simulink model "Model_3a_2015a"  (R2015a)
settings: Solver=ode45  StartTime=0.0  StopTime=10  RelTol=1e-3
undefined symbols (not defined in the file): c1, c2, K1, K2, K3, p1, Ts, wave
settings Model: CovModelRefEnable=off  Creator=s3blanch  LastModifiedBy=s3blanch
settings DataIOCC: SaveFormat=StructureWithTime
settings HardwareCC: ProdBitPerPointer=64  ProdLargestAtomicFloat=Float  ProdIntDivRoundTo=Zero  ProdEndianess=LittleEndian  ProdHWDeviceType=Specified
settings GRTTargetCC: GeneratePreprocessorConditionals=Use local settings

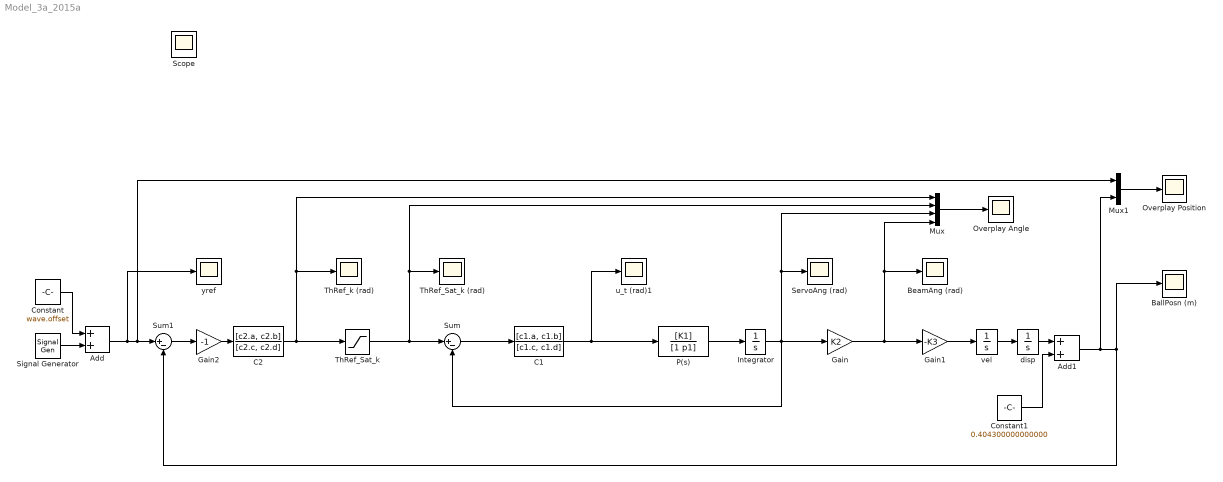
== system Model_3a_2015a ==
  " BeamAng (rad)" : Scope
      settings: YMin=-0.03886  YMax=0.03886  SaveName=BeamAng
  Add : Sum
  Add1 : Sum
  BallPosn (m) : Scope
      settings: YMin=-0.03732  YMax=0.33589  SaveName=BallPosn
  C1 : DiscreteTransferFcn  Numerator=[c1.a, c1.b]  Denominator=[c1.c, c1.d]  SampleTime=Ts
  C2 : DiscreteTransferFcn  Numerator=[c2.a, c2.b]  Denominator=[c2.c, c2.d]  SampleTime=Ts
  Constant : Constant  Value=wave.offset
  Constant1 : Constant  Value=0.404300000000000
  Gain : Gain  Gain=K2
  Gain1 : Gain  Gain=-K3
  Gain2 : Gain  Gain=-1
  Integrator : Integrator
  Mux : Mux
  Mux1 : Mux  Inputs=2
  Overplay Angle : Scope
      settings: TimeRange=25  YMin=-1.05154  YMax=1.20456
  Overplay Position : Scope
      settings: TimeRange=25  YMin=-0.03732  YMax=0.33589
  P(s) : TransferFcn  Numerator=[K1]  Denominator=[1 p1]
  ServoAng (rad) : Scope
      settings: YMin=-0.63804  YMax=0.63804  SaveName=ServoAng
  Signal Generator : SignalGenerator  WaveForm=square  Amplitude=-wave.amp  Frequency=0.2
  Sum : Sum  Inputs=|+-
  Sum1 : Sum  Inputs=|+-
  ThRef_Sat_k : Saturate  UpperLimit=0.7  LowerLimit=-0.7
  ThRef_Sat_k (rad) : Scope
      settings: YMin=-0.875  YMax=0.875  SaveName=ThRef
  ThRef_k (rad) : Scope
      settings: YMin=-1.05154  YMax=1.20456  SaveName=ref
  disp : Integrator
  u_t (rad)1 : Scope
      settings: YMin=-3.50155  YMax=2.92902  SaveName=u
  vel : Integrator
  yref : Scope
      settings: YMin=0.1275  YMax=0.2525  SaveName=yref
  Scope : Scope
      settings: YMin=-0.70238  YMax=0.70238
  wires:
  P(s)/1 -> Integrator/1
  Integrator/1 -> Gain/1, Sum/2, Mux/3, ServoAng (rad)/1
  Mux/1 -> Overplay Angle/1
  Sum/1 -> C1/1
  C1/1 -> P(s)/1, u_t (rad)1/1
  Gain1/1 -> vel/1
  vel/1 -> disp/1
  C2/1 -> Mux/1, ThRef_k (rad)/1, ThRef_Sat_k/1
  Mux1/1 -> Overplay Position/1
  Signal Generator/1 -> Add/2
  Constant/1 -> Add/1
  Add/1 -> Mux1/1, Sum1/1, yref/1
  Gain/1 -> Gain1/1, " BeamAng (rad)"/1, Mux/4
  ThRef_Sat_k/1 -> Sum/1, Mux/2, ThRef_Sat_k (rad)/1
  disp/1 -> Add1/1
  Add1/1 -> Mux1/2, Sum1/2, BallPosn (m)/1
  Constant1/1 -> Add1/2
  Gain2/1 -> C2/1
  Sum1/1 -> Gain2/1
